simulink model "LQR_control_XYmotion"  (R2025b)
settings: Solver=VariableStepAuto  StartTime=0.0  StopTime=10.0  RelTol=1e-3
values from neighbouring files (symbols this model uses):
  A_Mat = [ 0     1    0     0   0   0 ... (first row only)    [LQR_code_XYmotion.m]    (also in LQR_code_Xmotion.m = [ 0     1    0     0; LQR_control_AND_Plant2026.m = [ 0     1    0     0)
  B_Mat = [ 0    0 ... (first row only)    [LQR_code_XYmotion.m]    (also in LQR_code_Xmotion.m = [ 0; LQR_control_AND_Plant2026.m = [ 0)
  C_Mat = [ 1  0    0   0   0  0 ... (first row only)    [LQR_code_XYmotion.m]    (also in LQR_code_Xmotion.m = [ 1  0    0   0; LQR_control_AND_Plant2026.m = [ 1  0    0   0)
  D_Mat = [ 0    0 ... (first row only)    [LQR_code_XYmotion.m]
  K = lqr(A_Mat, B_Mat, Q, R)    [LQR_code_XYmotion.m]    (also in LQR_code_Xmotion.m; LQR_control_AND_Plant2026.m)
settings Model: Creator=Mahmoud Essam  LastModifiedBy=Mahmoud Essam

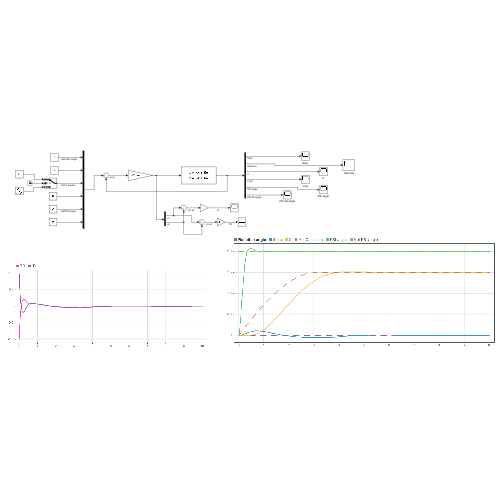
[thumbnail: Simulink's stored preview of the top-level diagram]
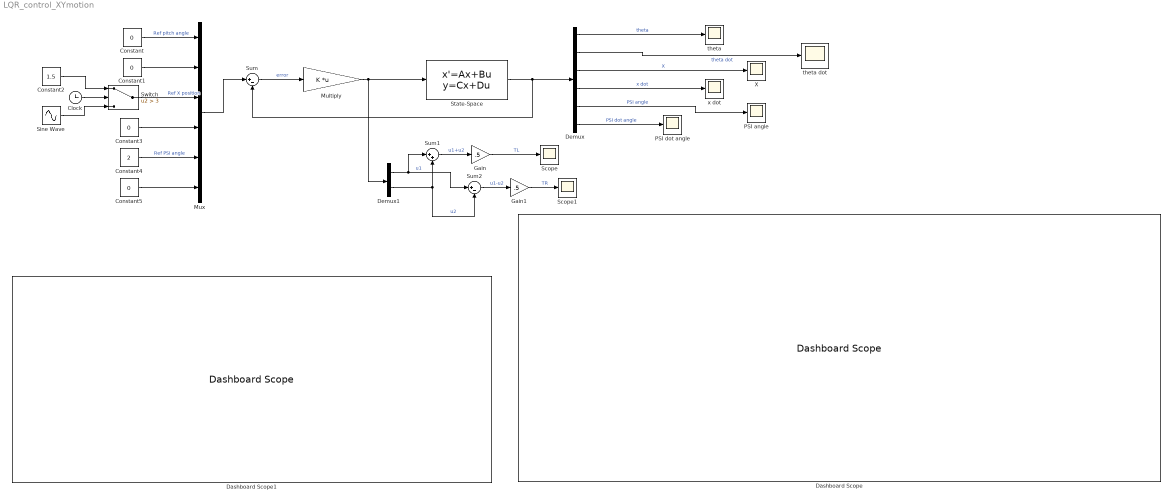
== system LQR_control_XYmotion ==
  " theta dot" : Scope
      settings: ActiveDisplayYMinimum=-22.999413149940512  ActiveDisplayYMaximum=55.548140907039681
  Clock : Clock
  Constant{,1,3,5} (4 alike) : Constant  Value=0
  Constant2 : Constant  Value=1.5
  Constant4 : Constant  Value=2
  Dashboard Scope : DashboardScope  FontColor=[0.0, 0.0, 0.0]
  Dashboard Scope1 : DashboardScope  FontColor=[0.0, 0.0, 0.0]
  Demux : Demux  Outputs=6
  Demux1 : Demux  Outputs=2
  Gain : Gain  Gain=.5
  Gain1 : Gain  Gain=.5
  Multiply : Gain  Gain=K  Multiplication=Matrix(K*u) (u vector)
  Mux : Mux  Inputs=6
  PSI angle : Scope
      settings: ActiveDisplayYMinimum=-1  ActiveDisplayYMaximum=1  DataLoggingVariableName=ScopeData4
  PSI dot angle : Scope
      settings: ActiveDisplayYMinimum=-1  ActiveDisplayYMaximum=1  DataLoggingVariableName=ScopeData5
  Scope : Scope
      settings: DataLoggingVariableName=ScopeData6
  Scope1 : Scope
      settings: DataLoggingVariableName=ScopeData7
  Sine Wave : Sin  Amplitude=1.5  Frequency=.5  SampleTime=0
  State-Space : StateSpace  A=A_Mat  B=B_Mat  C=C_Mat  D=D_Mat  InitialCondition=0
  Sum : Sum  Inputs=|+-
  Sum1 : Sum  Inputs=|++
  Sum2 : Sum  Inputs=|+-
  Switch : Switch  Criteria=u2 > Threshold  Threshold=3  SaturateOnIntegerOverflow=off  InputSameDT=off
  "X " : Scope
      settings: ActiveDisplayYMinimum=-1  ActiveDisplayYMaximum=1  DataLoggingVariableName=ScopeData2
  "theta " : Scope
      settings: ActiveDisplayYMinimum=-1  ActiveDisplayYMaximum=1
  x dot : Scope
      settings: ActiveDisplayYMinimum=-1  ActiveDisplayYMaximum=1  DataLoggingVariableName=ScopeData3
  wires:
  Demux/1 -> "theta "/1  "theta"
  Demux/2 -> " theta dot"/1  "theta dot"
  Multiply/1 -> Demux1/1, State-Space/1
  Demux/4 -> x dot/1  "x dot"
  Sum/1 -> Multiply/1  "error"
  State-Space/1 -> Sum/2, Demux/1
  Demux/3 -> "X "/1  "X"
  Mux/1 -> Sum/1
  Constant3/1 -> Mux/4
  Switch/1 -> Mux/3  "Ref X position"
  Constant1/1 -> Mux/2
  Constant/1 -> Mux/1  "Ref pitch angle"
  Clock/1 -> Switch/2
  Sine Wave/1 -> Switch/3
  Constant2/1 -> Switch/1
  Constant4/1 -> Mux/5  "Ref PSI angle"
  Constant5/1 -> Mux/6
  Demux/5 -> PSI angle/1  "PSI angle"
  Demux/6 -> PSI dot angle/1  "PSI dot angle"
  Demux1/1 -> Sum1/1, Sum2/1  "u1"
  Demux1/2 -> Sum2/2, Sum1/2  "u2"
  Sum1/1 -> Gain/1  "u1+u2"
  Sum2/1 -> Gain1/1  "u1-u2"
  Gain/1 -> Scope/1  "TL"
  Gain1/1 -> Scope1/1  "TR"
